simulink model "MSDRPrimaryLoop"  (R2021b)
settings: Solver=VariableStepAuto  StartTime=0.0  StopTime=250000  MaxStep=1  MinStep=0.01  RelTol=1e-3
undefined symbols (not defined in the file): a_f, A_free_PHX, a_g, A_h_PHX, beta, beta_t, bubbleGeneratorArea, bubbleGeneratorDh, bubbleGeneratorElevation, bubbleGeneratorLength, bubbleGeneratorVolume, bubbleSaturationLevel, bubbleSeparatorArea, bubbleSeparatorDiameter, bubbleSeparatorDo, bubbleSeparatorLength, bubbleSeparatorSlope, bypassRatio, C0, coreFlowArea, coreFuelVolume, coreLowerPlenumArea, coreLowerPlenumHydraulicDiameter, coreLowerPlenumLength, coreLowerPlenumVolume, coreUpperPlenumArea, coreUpperPlenumHydraulicDiameter, coreUpperPlenumLength, coreUpperPlenumVolume, coreVolume, cpGraphite, dissolusionRatio, dMin, dScale, dsmConst, DXeG, Fiss_factor, fuelChannelHydrualicDiameter, fuelChannelLength, fuelDepositRatio, fuelFraction, fuelGraphiteArea, fuelGraphiteHeatTransferCoefficient, gamma0, gamma1, gamma2, generatorDsm, graphiteKDiff, graphiteUnitCellThickness, initialIodineConcentration, InitialXeMolarConcentration, InjectionRatio, injectionRatio, iodineDecayConstant, IodineDecayConstant, iodineYield, kGraphite, kScale, Lam, lam ... (+59)
libraries: fl_lib x272, nesl_utility x105, SimscapeFluids_lib x24, slpidlib x1
(part 11 of 12)

== system MSDRPrimaryLoop/Reactor/CoreTH&Inerti/Core/CoreTH/CoreLinearNode3 ==
  note: Private model diameters are for MSDR only. These are based on the slab geometry and are not applicable to different reactor core design.
  note: Model with 1D simplified cylindrical quasi static heat transfer. Bi=0.26.
      | Refer to Nuclear Systems: 8.5.6. Or FHMT:5.5.2.
      | This is roughly ok for lumped analysis.
  GasRef : Inport
  2PModification : Subsystem  ReferencedSubsystem=TwoPhaseModification
      settings: PortSchema="{\"entries\":[{\"content\":{\"sides\":[{\"content\":{\"connectorIds\":[\"LConn1\"]},\"type\":\"ConnectorPlacement.EquallySpacedRectSide\",\"uuid\":\"7546b4b7-b669-49c8-8f27-f696391ea3ad\"},{\"content\":{\"connectorIds\":[\"RConn1\"],\"side\":\"RIGHT\"},\"type\":\"ConnectorPlacement.EquallySpacedRectSide\",\"uuid\":\"0e6176f2-177c-4327-bcfa-9a190fe9083f\"},{\"content\":{\"connectorIds\":[\"LConn2\",\"In1\"],\"side\":\"TOP\"},\"type\":\"ConnectorPlacement.EquallySpacedRectSide\",\"uuid\":\"16faf74c-4635-4009-a5b3-33dd03b625c6\"},{\"content\":{\"connectorIds\":[\"RConn2\"],\"side\":\"BOTTOM\"},\"type\":\"ConnectorPlacement.EquallySpacedRectSide\",\"uuid\":\"2081d73b-bb08-4ad9-b5c8-e48a4e9c4e20\"}]},\"type\":\"ConnectorPlacement.EquallySpacedConnector\",\"uuid\":\"243e4075-206b-4747-a8bc-b8f10d9a577f\"}],\"packageUris\":[\"http://schema.mathworks.com/mf0/Connector/R2020b\"],\"version\":\"1.0\"}"
  Conductive Heat Transfer1 : fl_lib/Thermal/Thermal Elements/Conductive Heat Transfer  area=CoreVolume/CoreLength*(1-FuelFraction) m^2  thickness=0.5*CoreLength/N_nodes m  th_cond=k_graphite W/(m*K)  T_specify=off  T_priority=None  T=0 K  T_nominal_specify=off  T_nominal_unit=K  T_nominal_value=1  Q_specify=off  Q_priority=None  Q=0 W  Q_nominal_specify=off  Q_nominal_unit=W  Q_nominal_value=1
  Conductive Heat Transfer2 : fl_lib/Thermal/Thermal Elements/Conductive Heat Transfer  area=CoreVolume/CoreLength*(1-FuelFraction) m^2  thickness=0.5*CoreLength/N_nodes m  th_cond=k_graphite W/(m*K)  T_specify=off  T_priority=None  T=0 K  T_nominal_specify=off  T_nominal_unit=K  T_nominal_value=1  Q_specify=off  Q_priority=None  Q=0 W  Q_nominal_specify=off  Q_nominal_unit=W  Q_nominal_value=1
  Conductive Heat Transfer3 : fl_lib/Thermal/Thermal Elements/Conductive Heat Transfer  area=FuelGraphiteArea/N_nodes m^2  thickness=0.5*UnitCellGraphiteThickness m  th_cond=k_graphite W/(m*K)  T_specify=off  T_priority=None  T=0 K  T_nominal_specify=off  T_nominal_unit=K  T_nominal_value=1  Q_specify=off  Q_priority=None  Q=0 W  Q_nominal_specify=off  Q_nominal_unit=W  Q_nominal_value=1
  Constant Volume Chamber (TL) : fl_lib/Thermal Liquid/Elements/Constant Volume Chamber (TL)  volume=0.001 m^3  num_ports=foundation.enum.num_ports.two  area_A=0.01 m^2  area_B=0.01 m^2  area_C=0.01 m^2  area_D=0.01 m^2  p_I_specify=on  p_I_priority=None  p_I=P0 Pa  p_I_nominal_specify=off  p_I_nominal_unit=MPa  p_I_nominal_value=1  T_I_specify=on  T_I_priority=None  T_I=T0 K  T_I_nominal_specify=off  T_I_nominal_unit=K  T_I_nominal_value=1  u_chamber_specify=on  u_chamber_priority=None  u_chamber=cpMSRE J/kg  u_chamber_nominal_specify=off  u_chamber_nominal_unit=kJ/kg  u_chamber_nominal_value=1  rho_specify=on  rho_priority=None  rho=nominalFuelDensity kg/m^3  rho_nominal_specify=off  rho_nominal_unit=kg/m^3  rho_nominal_value=1
      settings: SourceProductBaseCode=SS  LogSimulationData=on  InternalSimscapePortConfiguration="{\"Bottom\":[],\"Left\":[{\"id\":\"A\",\"label\":\"A\",\"type\":\"foundation.thermal_liquid.thermal_liquid\"},{\"id\":\"H\",\"label\":\"H\",\"type\":\"foundation.thermal.thermal\"}],\"Right\":[{\"id\":\"B\",\"label\":\"B\",\"type\":\"foundation.thermal_liquid.thermal_liquid\"}],\"Top\":[]}"
  Controlled Heat Flow Rate Source : fl_lib/Thermal/Thermal Sources/Controlled Heat Flow Rate Source
      settings: LogSimulationData=on
  Convective Heat Transfer : fl_lib/Thermal/Thermal Elements/Convective Heat Transfer  area=fuelGraphiteArea/N_nodes m^2  heat_tr_coeff=fuelGraphiteHeatTransferCoefficient W/(m^2*K)  T_specify=off  T_priority=None  T=0 K  T_nominal_specify=off  T_nominal_unit=K  T_nominal_value=1  Q_specify=off  Q_priority=None  Q=0 W  Q_nominal_specify=off  Q_nominal_unit=W  Q_nominal_value=1
  Fuel Deposited : fl_lib/Physical Signals/Functions/PS Gain  gain=FuelDepositRatio*CoreVolume/N_nodes m^3
  Grahite Deposited : fl_lib/Thermal/Thermal Sources/Controlled Heat Flow Rate Source
      settings: LogSimulationData=on
  Graphite Deposited : fl_lib/Physical Signals/Functions/PS Gain  gain=(1-FuelDepositRatio)*CoreVolume/N_nodes m^3
  Pipe (TL) : SimscapeFluids_lib/Thermal Liquid/Pipes & Fittings/Pipe (TL)  dynamic_compressibility=simscape.enum.onoff.on  inertia=simscape.enum.onoff.off  num_segments=1  pipe_length=fuelChannelLength/N_nodes m  area=coreFlowArea m^2  Dh=0.1128 m  wall_spec=fluids.thermal_liquid.pipes_fittings.enum.wall_spec.rigid  Dh_rigid=fuelChannelHydrualicDiameter m  wall_compliance=1.2e-6 m/MPa  wall_time_constant=0.01 s  elevation_spec=foundation.enum.constant_variable.constant  elevation_gain=fuelChannelLength/N_nodes m  g=9.82 m/s^2  pressure_loss_spec=fluids.thermal_liquid.pipes_fittings.enum.PressureLossSpec.Haaland  length_add=1 m  roughness=surfaceRoughness m  Re_friction_TLU=[400, 1000, 1500, 3000, 4000, 6000, 10000, 20000, 40000, 60000, 100000, 100000000]  friction_factor_TLU=[.264, .112, .071, .0417, .0387, .0268, .025, .0232, .0226, .022, .0214, .0214]  shape_factor=64  Re_lam=2000  Re_tur=4000  mdot_nominal=[.1, 1] kg/s  p_diff_nominal=[.001, .01] MPa  mdot_threshold=1e-6 kg/s  heat_transfer_spec=fluids.thermal_liquid.pipes_fittings.enum.HeatTransferSpec.Gnielinski  mdot_nominal_heat=[0.1, 10000] kg/s  T_in_nominal=[T0, T0] K  T_out_nominal=[T0, T0] K  p_in_nominal_heat=[.101325, .101325] MPa  T_wall_nominal=[T0+1, T0+1] K  a_coeff=0.023  b_Re_power=0.8  c_Pr_power=0.4  Nu_lam=3.66  Re_Colburn_TLU=[100, 150, 1000]  Colburn_factor_TLU=[.019, .013, .002]  Re_Nu_TLU=[100, 150, 1000]  Pr_Nu_TLU=[1, 10]  Nu_TLU=[3.72, 4.21; 3.75, 4.44; 4.21, 7.15]  T0_vec=T0 K  p0_vec=P0 Pa  mdot0=0.1 kg/s
      settings: SourceProductBaseCode=SH
  Temperature Sensor : fl_lib/Thermal/Thermal Sensors/Temperature Sensor
  Thermal Mass : fl_lib/Thermal/Thermal Elements/Thermal Mass  mass=CoreVolume*(1-FuelFraction)*rho_graphite/N_nodes kg  sp_heat=cp_graphite J/(K*kg)  T_specify=on  T_priority=High  T=T0 K  T_nominal_specify=off  T_nominal_unit=K  T_nominal_value=1  Q_specify=off  Q_priority=None  Q=0 W  Q_nominal_specify=off  Q_nominal_unit=W  Q_nominal_value=1
      settings: LogSimulationData=on
  Thermal Reference : fl_lib/Thermal/Thermal Elements/Thermal Reference
  Thermal Reference1 : fl_lib/Thermal/Thermal Elements/Thermal Reference
  Thermal Reference2 : fl_lib/Thermal/Thermal Elements/Thermal Reference
  Inlet : PMIOPort  Side=Left
  GraphiteA : PMIOPort  Port=2  Side=Left
  PowerDensity : PMIOPort  Port=3  Side=Left
  Outlet : PMIOPort  Port=4  Side=Right
  GraphiteB : PMIOPort  Port=5  Side=Right
  FuelTemp : PMIOPort  Port=6  Side=Right
  wires:
  GasRef/1 -> 2PModification/1
  connections:
  Grahite Deposited/LConn1 -- Conductive Heat Transfer3/RConn1 -- Conductive Heat Transfer2/RConn1 -- Thermal Mass/LConn1 -- Conductive Heat Transfer1/LConn1
  Graphite Deposited/LConn1 -- Fuel Deposited/LConn1 -- PowerDensity/RConn1
  Conductive Heat Transfer1/RConn1 -- GraphiteB/RConn1
  Grahite Deposited/RConn1 -- Graphite Deposited/RConn1
  GraphiteA/RConn1 -- Conductive Heat Transfer2/LConn1
  Controlled Heat Flow Rate Source/RConn2 -- Thermal Reference/LConn1
  Grahite Deposited/RConn2 -- Thermal Reference1/LConn1
  Fuel Deposited/RConn1 -- Controlled Heat Flow Rate Source/RConn1
  Outlet/RConn1 -- 2PModification/RConn1
  Temperature Sensor/RConn1 -- Thermal Reference2/LConn1
  Temperature Sensor/RConn2 -- FuelTemp/RConn1
  Inlet/RConn1 -- Constant Volume Chamber (TL)/LConn1
  Conductive Heat Transfer3/LConn1 -- Temperature Sensor/LConn1 -- Convective Heat Transfer/RConn1
  Constant Volume Chamber (TL)/LConn2 -- Convective Heat Transfer/LConn1 -- Controlled Heat Flow Rate Source/LConn1 -- Pipe (TL)/LConn2
  2PModification/RConn2 -- 2PModification/LConn1 -- Pipe (TL)/RConn1
  Constant Volume Chamber (TL)/RConn1 -- 2PModification/LConn2 -- Pipe (TL)/LConn1

== system MSDRPrimaryLoop/Reactor/CoreTH&Inerti/Core/CoreTH/PowerDensity ==
  note: This is a bit weird as the decay power is part of the total power.
      | I need to check the ratio of total power to decay power.
      | The 750MWth has to be refering to the...I don't know really.
  DecayFraction : Inport
  NeutronFraction : Inport  Port=2
  DecayPowerDensity : fl_lib/Physical Signals/Sources/PS Constant  constant=ReactorPower/CoreVolume*FuelInCoreRatio W/m^3
  PS Gain : fl_lib/Physical Signals/Functions/PS Gain  gain=3
  PS Min : fl_lib/Physical Signals/Nonlinear Operators/PS Min
      settings: SourceProductBaseCode=SS  InternalSimscapePortConfiguration="{\"Bottom\":[],\"Left\":[{\"id\":\"I1\",\"label\":\"\",\"type\":\"input\"},{\"id\":\"I2\",\"label\":\"\",\"type\":\"input\"}],\"Right\":[{\"id\":\"O\",\"label\":\"\",\"type\":\"output\"}],\"Top\":[]}"
  PS Product : fl_lib/Physical Signals/Functions/PS Product
  PS Product1 : fl_lib/Physical Signals/Functions/PS Product
  PowerDensity : fl_lib/Physical Signals/Sources/PS Constant  constant=ReactorPower/CoreVolume W/m^3
  Simulink-PS Converter : nesl_utility/Simulink-PS Converter  PhysicalDomain=network_engine_domain  SubClassName=ps_input  LeftPortType=input  RightPortType=output  PseudoPeriodic=off  Frequencies=[]  NoiseDistribution=none  NoiseParameters=[]  Unit=1  AffineConversion=off  FilteringAndDerivatives=provide  SimscapeFilterOrder=1  InputFilterTimeConstant=0.001  UdotUserProvided=0
      settings: SourceProductBaseCode=PW,SS
  Simulink-PS Converter1 : nesl_utility/Simulink-PS Converter  PhysicalDomain=network_engine_domain  SubClassName=ps_input  LeftPortType=input  RightPortType=output  PseudoPeriodic=off  Frequencies=[]  NoiseDistribution=none  NoiseParameters=[]  Unit=1  AffineConversion=off  FilteringAndDerivatives=provide  SimscapeFilterOrder=1  InputFilterTimeConstant=0.001  UdotUserProvided=0
      settings: SourceProductBaseCode=PW,SS
  TotalCorePower : fl_lib/Physical Signals/Functions/PS Add
  Conn1 : PMIOPort  Side=Right
  wires:
  DecayFraction/1 -> Simulink-PS Converter1/1
  NeutronFraction/1 -> Simulink-PS Converter/1
  connections:
  PS Product/RConn1 -- TotalCorePower/LConn1
  TotalCorePower/RConn1 -- PS Min/LConn2
  DecayPowerDensity/RConn1 -- PS Product1/LConn2
  PS Gain/RConn1 -- PS Min/LConn1
  Simulink-PS Converter/RConn1 -- PS Product/LConn2
  Simulink-PS Converter1/RConn1 -- PS Product1/LConn1
  PS Product1/RConn1 -- TotalCorePower/LConn2
  PS Min/RConn1 -- Conn1/RConn1
  PS Product/LConn1 -- PowerDensity/RConn1 -- PS Gain/LConn1

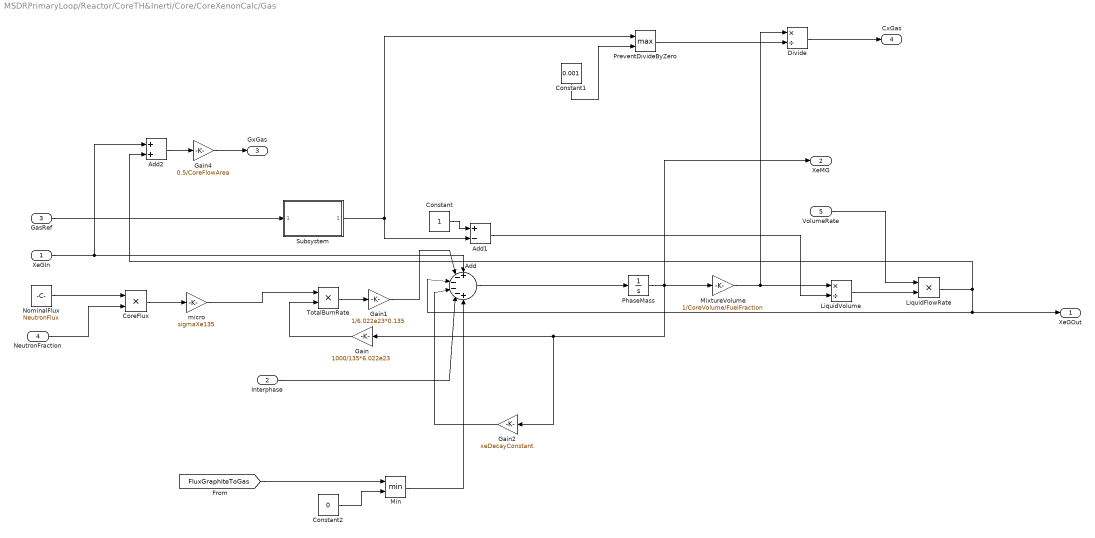
== system MSDRPrimaryLoop/Reactor/CoreTH&Inerti/Core/CoreXenonCalc/Gas ==
  XeGIn : Inport
  Interphase : Inport  Port=2
  GasRef : Inport  Port=3
  NeutronFraction : Inport  Port=4
  VolumeRate : Inport  Port=5
  Add : Sum  Inputs=+----+
  Add1 : Sum  Inputs=+-
  Add2 : Sum
  Constant : Constant
  Constant1 : Constant  Value=0.001
  Constant2 : Constant  Value=0
  CoreFlux : Product
  Divide : Product  Inputs=*/
  Gain : Gain  Gain=1000/135*6.022e23
  Gain1 : Gain  Gain=1/6.022e23*0.135
  Gain2 : Gain  Gain=xeDecayConstant
  Gain4 : Gain  Gain=0.5/CoreFlowArea
  LiquidFlowRate : Product
  LiquidVolume : Product  Inputs=*/
  Min : MinMax  Inputs=2
  MixtureVolume : Gain  Gain=1/CoreVolume/FuelFraction
  NominalFlux : Constant  Value=NeutronFlux
  PhaseMass : Integrator  LimitOutput=on  LowerSaturationLimit=0
  PreventDivideByZero : MinMax  Function=max  Inputs=2
  Subsystem : Subsystem  ReferencedSubsystem=GasToAlpha
  TotalBurnRate : Product
  micro : Gain  Gain=sigmaXe135
  XeGOut : Outport
  XeMG : Outport  Port=2
  GxGas : Outport  Port=3
  CxGas : Outport  Port=4
  wires:
  LiquidFlowRate/1 -> XeGOut/1, Add/3, Add2/2
  NominalFlux/1 -> CoreFlux/1
  LiquidVolume/1 -> LiquidFlowRate/2
  Add/1 -> PhaseMass/1
  CoreFlux/1 -> micro/1
  NeutronFraction/1 -> CoreFlux/2
  Constant/1 -> Add1/1
  Add1/1 -> LiquidVolume/2
  VolumeRate/1 -> LiquidFlowRate/1
  GasRef/1 -> Subsystem/1
  XeGIn/1 -> Add2/1, Add/1
  micro/1 -> TotalBurnRate/1
  Gain/1 -> TotalBurnRate/2
  TotalBurnRate/1 -> Gain1/1
  Gain1/1 -> Add/2
  Gain2/1 -> Add/4
  PhaseMass/1 -> XeMG/1, Gain2/1, Gain/1, MixtureVolume/1
  Interphase/1 -> Add/5
  Gain4/1 -> GxGas/1
  Add2/1 -> Gain4/1
  Constant1/1 -> PreventDivideByZero/2
  Divide/1 -> CxGas/1
  PreventDivideByZero/1 -> Divide/2
  MixtureVolume/1 -> LiquidVolume/1, Divide/1
  Subsystem/1 -> PreventDivideByZero/1, Add1/2
  [FluxGraphiteToGas] -> Min/1
  Min/1 -> Add/6
  Constant2/1 -> Min/2

== system MSDRPrimaryLoop/Reactor/CoreTH&Inerti/Core/CoreXenonCalc/InterphaseTranfser ==
  GxSalt : Inport
  NeutronFraction : Inport  Port=2
  GasRef : Inport  Port=3
  GxGas : Inport  Port=4
  CxSalt : Inport  Port=5
  T_f_ave : Inport  Port=6
  PLoss : Inport  Port=7
  CxGas : Inport  Port=8
  VolumeRate : Inport  Port=9
  Constant : Constant  Value=Dh
  Constant1 : Constant  Value=nominalNeutronFlux
  Constitutive : Subsystem
      settings: PortSchema="{\"entries\":[{\"content\":{\"sides\":[{\"content\":{\"connectorIds\":[\"In1\",\"LConn1\",\"In2\",\"In3\",\"In4\"]},\"type\":\"ConnectorPlacement.EquallySpacedRectSide\",\"uuid\":\"b30af6c3-7c55-4661-bc76-939f1c8a4177\"},{\"content\":{\"connectorIds\":[\"Out1\",\"Out2\",\"Out3\",\"Out4\",\"Out5\",\"Out6\",\"Out7\",\"Out8\",\"Out9\"],\"side\":\"RIGHT\"},\"type\":\"ConnectorPlacement.EquallySpacedRectSide\",\"uuid\":\"0b137634-5e01-4bd6-8381-72b0699f5835\"},{\"content\":{\"connectorIds\":[],\"side\":\"TOP\"},\"type\":\"ConnectorPlacement.EquallySpacedRectSide\",\"uuid\":\"06046061-3240-493e-a0a3-282c9541adae\"}]},\"type\":\"ConnectorPlacement.EquallySpacedConnector\",\"uuid\":\"b0591291-fd4b-4355-beaa-e569a19c4b12\"}],\"packageUris\":[\"http://schema.mathworks.com/mf0/Connector/R2020b\"],\"version\":\"1.0\"}"
  GraphiteInterchangeModel : Subsystem  mask{FuelGraphiteArea=FuelGraphiteArea, GraphiteVolume=CoreVolume*(1-FuelFraction), GraphitePorosity=0.1}
      mask prompts: FuelGraphiteArea "Fuel-Graphite Interface Area"; GraphiteVolume "Graphite Volume"; GraphitePorosity "Graphite Porosity"
  MixtureVolume : Gain  Gain=CoreVolume*FuelFraction
  Product : Product
  String Constant : StringConstant  String="\"upwards\""
  Subsystem : Subsystem  ReferencedSubsystem=kCalculation
      settings: PortSchema="{\"entries\":[{\"content\":{\"sides\":[{\"content\":{\"connectorIds\":[\"In2\",\"In3\",\"In4\",\"In5\",\"In6\",\"In7\",\"In1\"]},\"type\":\"ConnectorPlacement.EquallySpacedRectSide\",\"uuid\":\"002a6616-4b3b-4d3e-9efd-a784f6bbe134\"},{\"content\":{\"connectorIds\":[\"Out1\",\"Out2\"],\"side\":\"RIGHT\"},\"type\":\"ConnectorPlacement.EquallySpacedRectSide\",\"uuid\":\"da6acc14-6515-461b-8149-f4cbf493a4dd\"},{\"content\":{\"connectorIds\":[],\"side\":\"TOP\"},\"type\":\"ConnectorPlacement.EquallySpacedRectSide\",\"uuid\":\"939e49a4-f3cd-4ed3-a7a5-6bbefe0ae08a\"},{\"content\":{\"connectorIds\":[\"In8\"],\"side\":\"BOTTOM\"},\"type\":\"ConnectorPlacement.EquallySpacedRectSide\",\"uuid\":\"1ce110d7-af97-437a-ade8-04ae9fcd8383\"}]},\"type\":\"ConnectorPlacement.EquallySpacedConnector\",\"uuid\":\"8f0c794e-eb76-47c6-abaf-8e07cad1f307\"}],\"packageUris\":[\"http://schema.mathworks.com/mf0/Connector/R2020b\"],\"version\":\"1.0\"}"
  Subsystem1 : Subsystem  ReferencedSubsystem=GasToAlpha
  Transfer Term : MATLAB Function  TreatAsAtomicUnit=on
  Ref : PMIOPort  Side=Left
  TranfserRate : Outport
  XeMGraphite : Outport  Port=2
  tag scope: FluxGraphiteToGas=global, FluxGraphiteToSalt=global
  wires:
  Transfer Term/1(volRate) -> MixtureVolume/1
  MixtureVolume/1 -> TranfserRate/1
  Subsystem/2 -> Transfer Term/8(k)
  Subsystem/1 -> GraphiteInterchangeModel/5(dsm), Transfer Term/7(dsm)
  VolumeRate/1 -> Constitutive/3(VolumeRate)
  GasRef/1 -> Subsystem1/1
  Subsystem1/1 -> Constitutive/1(alpha), Transfer Term/3(alpha), GraphiteInterchangeModel/6(GasRef)
  Constitutive/1(ul) -> Transfer Term/4(ul), GraphiteInterchangeModel/7(ul)
  Constitutive/2(ug) -> Transfer Term/5(ug)
  Constitutive/3(K) -> Transfer Term/6(K)
  Constant/1 -> Subsystem/7, Constitutive/4(Diam)
  GxSalt/1 -> Transfer Term/1(GxS)
  GxGas/1 -> Transfer Term/2(GxG)
  CxGas/1 -> GraphiteInterchangeModel/4(CXeg)
  CxSalt/1 -> GraphiteInterchangeModel/1(CXef)
  T_f_ave/1 -> GraphiteInterchangeModel/3(Tempature)
  GraphiteInterchangeModel/3(Gas Diffusion Rate) -> [FluxGraphiteToGas]
  GraphiteInterchangeModel/1(Salt Diffusion Rate) -> [FluxGraphiteToSalt]
  GraphiteInterchangeModel/2(Xenon Mass In Graphite) -> XeMGraphite/1
  PLoss/1 -> Constitutive/2(PLoss)
  Constitutive/4(Re) -> Subsystem/2
  Constitutive/5(Sc) -> Subsystem/3
  Constitutive/6(Diff) -> Subsystem/4
  Constitutive/7(alphaC) -> Subsystem/5
  Constitutive/8(dsm) -> Subsystem/6
  Constitutive/9(f_m) -> Subsystem/1
  Constant1/1 -> Product/1
  NeutronFraction/1 -> Product/2
  Product/1 -> GraphiteInterchangeModel/2(phi)
  String Constant/1 -> Subsystem/8
  connections:
  Constitutive/LConn1 -- Ref/RConn1

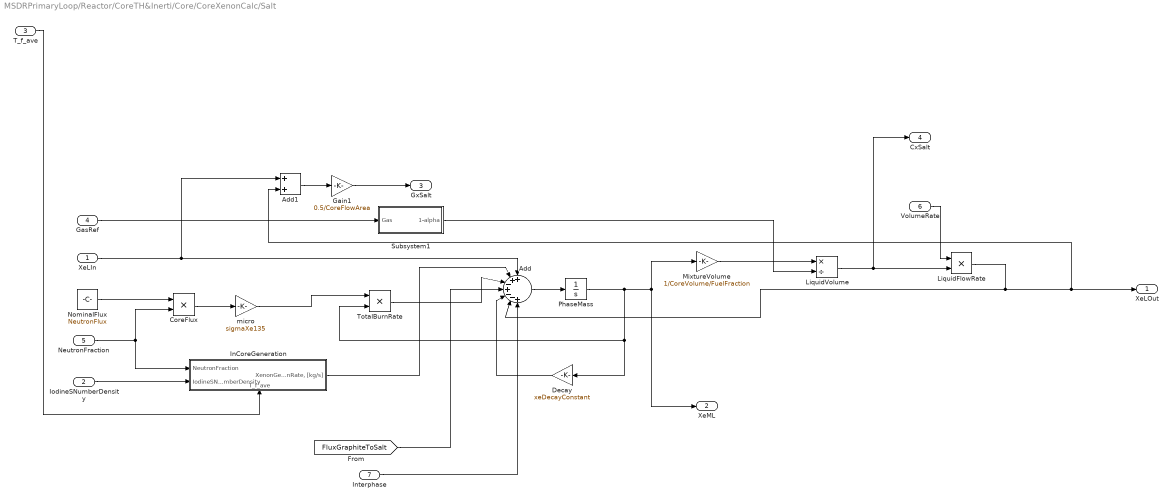
== system MSDRPrimaryLoop/Reactor/CoreTH&Inerti/Core/CoreXenonCalc/Salt ==
  XeLIn : Inport  PortDimensions=1
  IodineSNumberDensity : Inport  Port=2  PortDimensions=1
  T_f_ave : Inport  Port=3
  GasRef : Inport  Port=4  PortDimensions=1
  NeutronFraction : Inport  Port=5  PortDimensions=1
  VolumeRate : Inport  Port=6
  Interphase : Inport  Port=7
  Add : Sum  Inputs=++-+--+  InputSameDT=on
  Add1 : Sum
  CoreFlux : Product
  Decay : Gain  Gain=xeDecayConstant
  Gain1 : Gain  Gain=0.5/CoreFlowArea
  InCoreGeneration : Subsystem
      settings: PortSchema="{\"entries\":[{\"content\":{\"sides\":[{\"content\":{\"connectorIds\":[\"In1\",\"In2\"]},\"type\":\"ConnectorPlacement.EquallySpacedRectSide\",\"uuid\":\"cf58f9e2-4051-4ec0-bfd5-a375f3464f67\"},{\"content\":{\"connectorIds\":[\"Out1\"],\"side\":\"RIGHT\"},\"type\":\"ConnectorPlacement.EquallySpacedRectSide\",\"uuid\":\"cf475b22-0422-4ebc-b148-ab559744c6ba\"},{\"content\":{\"connectorIds\":[],\"side\":\"TOP\"},\"type\":\"ConnectorPlacement.EquallySpacedRectSide\",\"uuid\":\"15cc78ce-ee79-4f49-b098-b77c0b2a8ba1\"},{\"content\":{\"connectorIds\":[\"In3\"],\"side\":\"BOTTOM\"},\"type\":\"ConnectorPlacement.EquallySpacedRectSide\",\"uuid\":\"64f5be1f-19d6-4b5f-ac24-c41659a6a539\"}]},\"type\":\"ConnectorPlacement.EquallySpacedConnector\",\"uuid\":\"1fb1607a-ceed-4d70-a511-7b706be0d7ea\"}],\"packageUris\":[\"http://schema.mathworks.com/mf0/Connector/R2020b\"],\"version\":\"1.0\"}"
  LiquidFlowRate : Product
  LiquidVolume : Product  Inputs=*/
  MixtureVolume : Gain  Gain=1/CoreVolume/FuelFraction
  NominalFlux : Constant  Value=NeutronFlux
  PhaseMass : Integrator  LimitOutput=on  LowerSaturationLimit=0
  Subsystem1 : Subsystem
  TotalBurnRate : Product
  micro : Gain  Gain=sigmaXe135
  XeLOut : Outport  PortDimensions=1
  XeML : Outport  Port=2  PortDimensions=1
  GxSalt : Outport  Port=3
  CxSalt : Outport  Port=4
  wires:
  LiquidFlowRate/1 -> Add/6, Add1/2, XeLOut/1
  IodineSNumberDensity/1 -> InCoreGeneration/2(IodineSNumberDensity)
  NominalFlux/1 -> CoreFlux/1
  LiquidVolume/1 -> CxSalt/1, LiquidFlowRate/2
  Add/1 -> PhaseMass/1
  CoreFlux/1 -> micro/1
  NeutronFraction/1 -> InCoreGeneration/1(NeutronFraction), CoreFlux/2
  MixtureVolume/1 -> LiquidVolume/1
  VolumeRate/1 -> LiquidFlowRate/1
  T_f_ave/1 -> InCoreGeneration/3(T_f_ave)
  XeLIn/1 -> Add1/1, Add/1
  micro/1 -> TotalBurnRate/1
  PhaseMass/1 -> TotalBurnRate/2, Decay/1, XeML/1, MixtureVolume/1
  Decay/1 -> Add/5
  GasRef/1 -> Subsystem1/1(Gas)
  Subsystem1/1(1-alpha) -> LiquidVolume/2
  [FluxGraphiteToSalt] -> Add/4
  InCoreGeneration/1("XenonGenerationRate, [kg/s]") -> Add/2
  TotalBurnRate/1 -> Add/3
  Interphase/1 -> Add/7
  Gain1/1 -> GxSalt/1
  Add1/1 -> Gain1/1

== system MSDRPrimaryLoop/Reactor/CoreTH&Inerti/Core/SolubilityReduction/If Action Subsystem ==
  GasLeft : Inport
  Action Port : ActionPort  ActionPortLabel=if(u1 > 0)
  Constant : Constant  Value=dissolusionRatio
  Gain : Gain
  GasOut : Outport
  AbsorbedGas : Outport  Port=2
  wires:
  GasLeft/1 -> GasOut/1
  Constant/1 -> Gain/1
  Gain/1 -> AbsorbedGas/1

== system MSDRPrimaryLoop/Reactor/CoreTH&Inerti/Core/SolubilityReduction/If Action Subsystem1 ==
  GasIn : Inport
  Action Port : ActionPort  ActionPortLabel=else
  Constant : Constant  Value=0
  GasOut : Outport
  AbsorbedGas : Outport  Port=2
  wires:
  GasIn/1 -> AbsorbedGas/1
  Constant/1 -> GasOut/1

== system MSDRPrimaryLoop/Reactor/CoreTH&Inerti/Core/Subsystem1/GasCalc ==
  GasIn : Inport
  Add : Sum  Inputs=+-
  GasExpansion : Subsystem  ReferencedSubsystem=GasExpansion
      settings: PortSchema="{\"entries\":[{\"content\":{\"sides\":[{\"content\":{\"connectorIds\":[\"LConn1\",\"In1\"]},\"type\":\"ConnectorPlacement.EquallySpacedRectSide\",\"uuid\":\"50c89675-cb8a-4964-af62-cb2014507b1d\"},{\"content\":{\"connectorIds\":[\"RConn1\",\"Out1\"],\"side\":\"RIGHT\"},\"type\":\"ConnectorPlacement.EquallySpacedRectSide\",\"uuid\":\"6b3adc78-0be5-4682-9da0-6fd41ffc4e71\"},{\"content\":{\"connectorIds\":[],\"side\":\"TOP\"},\"type\":\"ConnectorPlacement.EquallySpacedRectSide\",\"uuid\":\"5158b46f-a496-48e4-90d6-6c6dcc9e237b\"}]},\"type\":\"ConnectorPlacement.EquallySpacedConnector\",\"uuid\":\"7ff0188e-dc19-44a0-a8cf-bde33949414f\"}],\"packageUris\":[\"http://schema.mathworks.com/mf0/Connector/R2020b\"],\"version\":\"1.0\"}"
  Integrator : Integrator  InitialCondition=injectionRatio*CoreVolume*FuelFraction
  PS-Simulink Converter : nesl_utility/PS-Simulink Converter  PhysicalDomain=network_engine_domain  SubClassName=ps_output  LeftPortType=input  RightPortType=output  PseudoPeriodic=off  Frequencies=[]  Unit=inherit  AffineConversion=off
      settings: SourceProductBaseCode=PW,SS
  Product : Product
  VolumeToVoid : Gain  Gain=1/(CoreVolume*FuelFraction)
  VolumeRate : PMIOPort  Side=Left
  Ref1 : PMIOPort  Port=2  Side=Right
  Ref2 : PMIOPort  Port=3  Side=Right
  GasOut : Outport
  wires:
  VolumeToVoid/1 -> GasExpansion/1, Add/2
  Integrator/1 -> VolumeToVoid/1
  GasIn/1 -> Add/1
  Add/1 -> Product/1
  Product/1 -> Integrator/1
  PS-Simulink Converter/1 -> Product/2
  GasExpansion/1 -> GasOut/1
  connections:
  PS-Simulink Converter/LConn1 -- VolumeRate/RConn1
  GasExpansion/LConn1 -- Ref1/RConn1
  GasExpansion/RConn1 -- Ref2/RConn1

== system MSDRPrimaryLoop/Reactor/CoreTH&Inerti/Core/Subsystem2/SolubilityModificationPrescribed ==
  note: The idea is that when the dissolved gas comes back out, it is saturated with xenon because of the super efficiency removal of micro bubbles. The gain factor is used to adjust the concentration of the bubbles to less than saturation.
  XeIn : Inport
  GasIn : Inport  Port=2
  AbsorbedOut : Inport  Port=3
  Temperature : Inport  Port=4
  Add : Sum
  Add1 : Sum
  AddedBackGas : Sum
  Constant : Constant
  Demux : Demux  Outputs=2
  Divide : Product  Inputs=**/
  Divide1 : Product  Inputs=*/
  Divide2 : Product  Inputs=*/
  Gain : Gain  Gain=bubbleSaturationLevel
  KScale : Subsystem  ReferencedSubsystem=KScale
  Mux : Mux  Inputs=2
  XeOut : Outport
  GasOut : Outport  Port=2
  wires:
  GasIn/1 -> AddedBackGas/1
  AbsorbedOut/1 -> Divide2/1, AddedBackGas/2
  AddedBackGas/1 -> GasOut/1
  XeIn/1 -> Demux/1
  Mux/1 -> XeOut/1
  Temperature/1 -> KScale/1
  KScale/1 -> Divide2/2
  Constant/1 -> Add/2
  Divide2/1 -> Gain/1
  Add/1 -> Divide1/2, Divide/3
  Demux/1 -> Divide/1, Divide1/1
  Demux/2 -> Add1/1
  Divide/1 -> Add1/2
  Add1/1 -> Mux/2
  Divide1/1 -> Mux/1
  Gain/1 -> Add/1, Divide/2

== system MSDRPrimaryLoop/Reactor/CoreTH&Inerti/Core/Subsystem2/Subsystem2 ==
  note: Switch between prescibed concentration and near-zero based on whether bubbles are present.
  XeIn : Inport
  GasIn : Inport  Port=2
  AbsorbedOut : Inport  Port=3
  Temperature : Inport  Port=4
  ModeSwitch : Inport  Port=5
  If : If
  If Action Subsystem : Subsystem  TreatAsAtomicUnit=on
  If Action Subsystem1 : Subsystem  TreatAsAtomicUnit=on
  Merge : Merge
  Merge1 : Merge
  GasOut : Outport
  XeOut : Outport  Port=2
  wires:
  ModeSwitch/1 -> If/1
  If/1 -> If Action Subsystem/Action
  If/2 -> If Action Subsystem1/Action
  AbsorbedOut/1 -> If Action Subsystem1/2(AbsorbedOut), If Action Subsystem/2(AbsorbedOut)
  GasIn/1 -> If Action Subsystem1/1(GasIn), If Action Subsystem/1(GasIn)
  XeIn/1 -> If Action Subsystem/3(XeIn), If Action Subsystem1/3(XeIn)
  Merge/1 -> GasOut/1
  If Action Subsystem/1(GasOut) -> Merge/1
  If Action Subsystem1/1(GasOut) -> Merge/2
  If Action Subsystem/2(XeOut) -> Merge1/1
  If Action Subsystem1/2(XeOut) -> Merge1/2
  Merge1/1 -> XeOut/1
  Temperature/1 -> If Action Subsystem1/4(Temperature)

== system MSDRPrimaryLoop/Reactor/CoreTH&Inerti/LowerPlenum/XenonCalc/Gas ==
  XeGIn : Inport
  Interphase : Inport  Port=2
  GasRef : Inport  Port=3
  VolumeRate : Inport  Port=4
  Add : Sum  Inputs=+---
  Add1 : Sum  Inputs=+-
  Add2 : Sum
  Constant : Constant
  Gain2 : Gain  Gain=xeDecayConstant
  Gain4 : Gain  Gain=0.5/Area
  LiquidFlowRate : Product
  LiquidVolume : Product  Inputs=*/
  MixtureVolume : Gain  Gain=1/Volume
  PhaseMass : Integrator  LimitOutput=on  LowerSaturationLimit=0
  Subsystem : Subsystem  ReferencedSubsystem=GasToAlpha
  XeGOut : Outport
  GxGas : Outport  Port=2
  wires:
  LiquidFlowRate/1 -> XeGOut/1, Add2/2, Add/3
  Subsystem/1 -> Add1/2
  LiquidVolume/1 -> LiquidFlowRate/2
  Add/1 -> PhaseMass/1
  Constant/1 -> Add1/1
  MixtureVolume/1 -> LiquidVolume/1
  Add1/1 -> LiquidVolume/2
  VolumeRate/1 -> LiquidFlowRate/1
  GasRef/1 -> Subsystem/1
  XeGIn/1 -> Add/1, Add2/1
  Gain2/1 -> Add/4
  PhaseMass/1 -> Gain2/1, MixtureVolume/1
  Gain4/1 -> GxGas/1
  Add2/1 -> Gain4/1
  Interphase/1 -> Add/2

== system MSDRPrimaryLoop/Reactor/CoreTH&Inerti/LowerPlenum/XenonCalc/InterphaseTranfser ==
  note: This local to volume isn't strick. Either add an integral or reduce the length of the node if variation is large.
  GxSalt : Inport
  GasRef : Inport  Port=2
  GxGas : Inport  Port=3
  PLoss : Inport  Port=4
  VolumeRate : Inport  Port=5
  Constant : Constant  Value=Dh
  Constitutive : Subsystem
      settings: PortSchema="{\"entries\":[{\"content\":{\"sides\":[{\"content\":{\"connectorIds\":[\"In1\",\"LConn1\",\"In2\",\"In3\",\"In4\"]},\"type\":\"ConnectorPlacement.EquallySpacedRectSide\",\"uuid\":\"b30af6c3-7c55-4661-bc76-939f1c8a4177\"},{\"content\":{\"connectorIds\":[\"Out1\",\"Out2\",\"Out3\",\"Out4\",\"Out5\",\"Out6\",\"Out7\",\"Out8\",\"Out9\"],\"side\":\"RIGHT\"},\"type\":\"ConnectorPlacement.EquallySpacedRectSide\",\"uuid\":\"0b137634-5e01-4bd6-8381-72b0699f5835\"},{\"content\":{\"connectorIds\":[],\"side\":\"TOP\"},\"type\":\"ConnectorPlacement.EquallySpacedRectSide\",\"uuid\":\"06046061-3240-493e-a0a3-282c9541adae\"}]},\"type\":\"ConnectorPlacement.EquallySpacedConnector\",\"uuid\":\"b0591291-fd4b-4355-beaa-e569a19c4b12\"}],\"packageUris\":[\"http://schema.mathworks.com/mf0/Connector/R2020b\"],\"version\":\"1.0\"}"
  MixtureVolume : Gain  Gain=Volume
  String Constant : StringConstant  String="\"upwards\""
  Subsystem : Subsystem  ReferencedSubsystem=kCalculation
      settings: PortSchema="{\"entries\":[{\"content\":{\"sides\":[{\"content\":{\"connectorIds\":[\"In2\",\"In3\",\"In4\",\"In5\",\"In6\",\"In7\",\"In1\"]},\"type\":\"ConnectorPlacement.EquallySpacedRectSide\",\"uuid\":\"002a6616-4b3b-4d3e-9efd-a784f6bbe134\"},{\"content\":{\"connectorIds\":[\"Out1\",\"Out2\"],\"side\":\"RIGHT\"},\"type\":\"ConnectorPlacement.EquallySpacedRectSide\",\"uuid\":\"da6acc14-6515-461b-8149-f4cbf493a4dd\"},{\"content\":{\"connectorIds\":[],\"side\":\"TOP\"},\"type\":\"ConnectorPlacement.EquallySpacedRectSide\",\"uuid\":\"939e49a4-f3cd-4ed3-a7a5-6bbefe0ae08a\"},{\"content\":{\"connectorIds\":[\"In8\"],\"side\":\"BOTTOM\"},\"type\":\"ConnectorPlacement.EquallySpacedRectSide\",\"uuid\":\"df8afac6-b18f-4ec8-9e08-eea5226bf274\"}]},\"type\":\"ConnectorPlacement.EquallySpacedConnector\",\"uuid\":\"8f0c794e-eb76-47c6-abaf-8e07cad1f307\"}],\"packageUris\":[\"http://schema.mathworks.com/mf0/Connector/R2020b\"],\"version\":\"1.0\"}"
  Subsystem1 : Subsystem  ReferencedSubsystem=GasToAlpha
  Transfer Term : MATLAB Function  TreatAsAtomicUnit=on
  Ref : PMIOPort  Side=Left
  TranfserRate : Outport
  wires:
  Transfer Term/1(volRate) -> MixtureVolume/1
  MixtureVolume/1 -> TranfserRate/1
  VolumeRate/1 -> Constitutive/3(VolumeRate)
  GasRef/1 -> Subsystem1/1
  Subsystem1/1 -> Constitutive/1(alpha), Transfer Term/3(alpha)
  Constitutive/1(ul) -> Transfer Term/4(ul)
  Constitutive/2(ug) -> Transfer Term/5(ug)
  Constitutive/3(K) -> Transfer Term/6(K)
  Constant/1 -> Subsystem/7, Constitutive/4(Diam)
  GxSalt/1 -> Transfer Term/1(GxS)
  GxGas/1 -> Transfer Term/2(GxG)
  Constitutive/9(f_m) -> Subsystem/1
  Constitutive/4(Re) -> Subsystem/2
  Constitutive/5(Sc) -> Subsystem/3
  Constitutive/7(alphaC) -> Subsystem/5
  Subsystem/1 -> Transfer Term/7(dsm)
  Subsystem/2 -> Transfer Term/8(k)
  PLoss/1 -> Constitutive/2(PLoss)
  Constitutive/8(dsm) -> Subsystem/6
  Constitutive/6(Diff) -> Subsystem/4
  String Constant/1 -> Subsystem/8
  connections:
  Ref/RConn1 -- Constitutive/LConn1

== system MSDRPrimaryLoop/Reactor/CoreTH&Inerti/LowerPlenum/XenonCalc/Salt ==
  XeLIn : Inport  PortDimensions=1
  IodineSNumberDensity : Inport  Port=2  PortDimensions=1
  T_f_ave : Inport  Port=3
  GasRef : Inport  Port=4  PortDimensions=1
  VolumeRate : Inport  Port=5
  Interphase : Inport  Port=6
  Add : Sum  Inputs=+++--  InputSameDT=on
  Add1 : Sum
  Decay : Gain  Gain=xeDecayConstant
  Gain1 : Gain  Gain=0.5/Area
  InPipeGeneration : Subsystem
      settings: PortSchema="{\"entries\":[{\"content\":{\"sides\":[{\"content\":{\"connectorIds\":[\"In1\"]},\"type\":\"ConnectorPlacement.EquallySpacedRectSide\",\"uuid\":\"cf58f9e2-4051-4ec0-bfd5-a375f3464f67\"},{\"content\":{\"connectorIds\":[\"Out1\"],\"side\":\"RIGHT\"},\"type\":\"ConnectorPlacement.EquallySpacedRectSide\",\"uuid\":\"cf475b22-0422-4ebc-b148-ab559744c6ba\"},{\"content\":{\"connectorIds\":[],\"side\":\"TOP\"},\"type\":\"ConnectorPlacement.EquallySpacedRectSide\",\"uuid\":\"15cc78ce-ee79-4f49-b098-b77c0b2a8ba1\"},{\"content\":{\"connectorIds\":[\"In2\"],\"side\":\"BOTTOM\"},\"type\":\"ConnectorPlacement.EquallySpacedRectSide\",\"uuid\":\"64f5be1f-19d6-4b5f-ac24-c41659a6a539\"}]},\"type\":\"ConnectorPlacement.EquallySpacedConnector\",\"uuid\":\"1fb1607a-ceed-4d70-a511-7b706be0d7ea\"}],\"packageUris\":[\"http://schema.mathworks.com/mf0/Connector/R2020b\"],\"version\":\"1.0\"}"
  LiquidFlowRate : Product
  LiquidVolume : Product  Inputs=*/
  MixtureVolume : Gain  Gain=1/Volume
  PhaseMass : Integrator  LimitOutput=on  LowerSaturationLimit=0
  Subsystem1 : Subsystem
  XeLOut : Outport  PortDimensions=1
  GxSalt : Outport  Port=2
  wires:
  LiquidFlowRate/1 -> Add/5, XeLOut/1, Add1/2
  IodineSNumberDensity/1 -> InPipeGeneration/1(IodineSNumberDensity)
  LiquidVolume/1 -> LiquidFlowRate/2
  Add/1 -> PhaseMass/1
  MixtureVolume/1 -> LiquidVolume/1
  VolumeRate/1 -> LiquidFlowRate/1
  T_f_ave/1 -> InPipeGeneration/2(T_f_ave)
  PhaseMass/1 -> Decay/1, MixtureVolume/1
  GasRef/1 -> Subsystem1/1(Gas)
  Subsystem1/1(1-alpha) -> LiquidVolume/2
  InPipeGeneration/1("XenonGenerationRate, [kg/s]") -> Add/2
  XeLIn/1 -> Add1/1, Add/1
  Add1/1 -> Gain1/1
  Gain1/1 -> GxSalt/1
  Interphase/1 -> Add/3
  Decay/1 -> Add/4

== system MSDRPrimaryLoop/Reactor/CoreTH&Inerti/UpperPlenum/XenonCalc/Gas ==
  XeGIn : Inport
  Interphase : Inport  Port=2
  GasRef : Inport  Port=3
  VolumeRate : Inport  Port=4
  Add : Sum  Inputs=+---
  Add1 : Sum  Inputs=+-
  Add2 : Sum
  Constant : Constant
  Gain2 : Gain  Gain=xeDecayConstant
  Gain4 : Gain  Gain=0.5/Area
  LiquidFlowRate : Product
  LiquidVolume : Product  Inputs=*/
  MixtureVolume : Gain  Gain=1/Volume
  PhaseMass : Integrator  LimitOutput=on  LowerSaturationLimit=0
  Subsystem : Subsystem  ReferencedSubsystem=GasToAlpha
  XeGOut : Outport
  GxGas : Outport  Port=2
  wires:
  LiquidFlowRate/1 -> XeGOut/1, Add2/2, Add/3
  Subsystem/1 -> Add1/2
  LiquidVolume/1 -> LiquidFlowRate/2
  Add/1 -> PhaseMass/1
  Constant/1 -> Add1/1
  MixtureVolume/1 -> LiquidVolume/1
  Add1/1 -> LiquidVolume/2
  VolumeRate/1 -> LiquidFlowRate/1
  GasRef/1 -> Subsystem/1
  XeGIn/1 -> Add/1, Add2/1
  Gain2/1 -> Add/4
  PhaseMass/1 -> Gain2/1, MixtureVolume/1
  Gain4/1 -> GxGas/1
  Add2/1 -> Gain4/1
  Interphase/1 -> Add/2

== system MSDRPrimaryLoop/Reactor/CoreTH&Inerti/UpperPlenum/XenonCalc/InterphaseTranfser ==
  note: This local to volume isn't strick. Either add an integral or reduce the length of the node if variation is large.
  GxSalt : Inport
  GasRef : Inport  Port=2
  GxGas : Inport  Port=3
  PLoss : Inport  Port=4
  VolumeRate : Inport  Port=5
  Constant : Constant  Value=Dh
  Constitutive : Subsystem
      settings: PortSchema="{\"entries\":[{\"content\":{\"sides\":[{\"content\":{\"connectorIds\":[\"In1\",\"LConn1\",\"In2\",\"In3\",\"In4\"]},\"type\":\"ConnectorPlacement.EquallySpacedRectSide\",\"uuid\":\"b30af6c3-7c55-4661-bc76-939f1c8a4177\"},{\"content\":{\"connectorIds\":[\"Out1\",\"Out2\",\"Out3\",\"Out4\",\"Out5\",\"Out6\",\"Out7\",\"Out8\",\"Out9\"],\"side\":\"RIGHT\"},\"type\":\"ConnectorPlacement.EquallySpacedRectSide\",\"uuid\":\"0b137634-5e01-4bd6-8381-72b0699f5835\"},{\"content\":{\"connectorIds\":[],\"side\":\"TOP\"},\"type\":\"ConnectorPlacement.EquallySpacedRectSide\",\"uuid\":\"06046061-3240-493e-a0a3-282c9541adae\"}]},\"type\":\"ConnectorPlacement.EquallySpacedConnector\",\"uuid\":\"b0591291-fd4b-4355-beaa-e569a19c4b12\"}],\"packageUris\":[\"http://schema.mathworks.com/mf0/Connector/R2020b\"],\"version\":\"1.0\"}"
  MixtureVolume : Gain  Gain=Volume
  String Constant : StringConstant  String="\"upwards\""
  Subsystem : Subsystem  ReferencedSubsystem=kCalculation
      settings: PortSchema="{\"entries\":[{\"content\":{\"sides\":[{\"content\":{\"connectorIds\":[\"In2\",\"In3\",\"In4\",\"In5\",\"In6\",\"In7\",\"In1\"]},\"type\":\"ConnectorPlacement.EquallySpacedRectSide\",\"uuid\":\"002a6616-4b3b-4d3e-9efd-a784f6bbe134\"},{\"content\":{\"connectorIds\":[\"Out1\",\"Out2\"],\"side\":\"RIGHT\"},\"type\":\"ConnectorPlacement.EquallySpacedRectSide\",\"uuid\":\"da6acc14-6515-461b-8149-f4cbf493a4dd\"},{\"content\":{\"connectorIds\":[],\"side\":\"TOP\"},\"type\":\"ConnectorPlacement.EquallySpacedRectSide\",\"uuid\":\"939e49a4-f3cd-4ed3-a7a5-6bbefe0ae08a\"},{\"content\":{\"connectorIds\":[\"In8\"],\"side\":\"BOTTOM\"},\"type\":\"ConnectorPlacement.EquallySpacedRectSide\",\"uuid\":\"3faad216-807b-414f-aa2c-73b0ff13b323\"}]},\"type\":\"ConnectorPlacement.EquallySpacedConnector\",\"uuid\":\"8f0c794e-eb76-47c6-abaf-8e07cad1f307\"}],\"packageUris\":[\"http://schema.mathworks.com/mf0/Connector/R2020b\"],\"version\":\"1.0\"}"
  Subsystem1 : Subsystem  ReferencedSubsystem=GasToAlpha
  Transfer Term : MATLAB Function  TreatAsAtomicUnit=on
  Ref : PMIOPort  Side=Left
  TranfserRate : Outport
  wires:
  Transfer Term/1(volRate) -> MixtureVolume/1
  MixtureVolume/1 -> TranfserRate/1
  VolumeRate/1 -> Constitutive/3(VolumeRate)
  GasRef/1 -> Subsystem1/1
  Subsystem1/1 -> Constitutive/1(alpha), Transfer Term/3(alpha)
  Constitutive/1(ul) -> Transfer Term/4(ul)
  Constitutive/2(ug) -> Transfer Term/5(ug)
  Constant/1 -> Subsystem/7, Constitutive/4(Diam)
  GxSalt/1 -> Transfer Term/1(GxS)
  GxGas/1 -> Transfer Term/2(GxG)
  Subsystem/1 -> Transfer Term/7(dsm)
  Subsystem/2 -> Transfer Term/8(k)
  PLoss/1 -> Constitutive/2(PLoss)
  Constitutive/4(Re) -> Subsystem/2
  Constitutive/3(K) -> Transfer Term/6(K)
  Constitutive/5(Sc) -> Subsystem/3
  Constitutive/6(Diff) -> Subsystem/4
  Constitutive/7(alphaC) -> Subsystem/5
  Constitutive/8(dsm) -> Subsystem/6
  Constitutive/9(f_m) -> Subsystem/1
  String Constant/1 -> Subsystem/8
  connections:
  Constitutive/LConn1 -- Ref/RConn1

== system MSDRPrimaryLoop/Reactor/CoreTH&Inerti/UpperPlenum/XenonCalc/Salt ==
  XeLIn : Inport  PortDimensions=1
  IodineSNumberDensity : Inport  Port=2  PortDimensions=1
  T_f_ave : Inport  Port=3
  GasRef : Inport  Port=4  PortDimensions=1
  VolumeRate : Inport  Port=5
  Interphase : Inport  Port=6
  Add : Sum  Inputs=+++--  InputSameDT=on
  Add1 : Sum
  Decay : Gain  Gain=xeDecayConstant
  Gain1 : Gain  Gain=0.5/Area
  InPipeGeneration : Subsystem
      settings: PortSchema="{\"entries\":[{\"content\":{\"sides\":[{\"content\":{\"connectorIds\":[\"In1\"]},\"type\":\"ConnectorPlacement.EquallySpacedRectSide\",\"uuid\":\"cf58f9e2-4051-4ec0-bfd5-a375f3464f67\"},{\"content\":{\"connectorIds\":[\"Out1\"],\"side\":\"RIGHT\"},\"type\":\"ConnectorPlacement.EquallySpacedRectSide\",\"uuid\":\"cf475b22-0422-4ebc-b148-ab559744c6ba\"},{\"content\":{\"connectorIds\":[],\"side\":\"TOP\"},\"type\":\"ConnectorPlacement.EquallySpacedRectSide\",\"uuid\":\"15cc78ce-ee79-4f49-b098-b77c0b2a8ba1\"},{\"content\":{\"connectorIds\":[\"In2\"],\"side\":\"BOTTOM\"},\"type\":\"ConnectorPlacement.EquallySpacedRectSide\",\"uuid\":\"64f5be1f-19d6-4b5f-ac24-c41659a6a539\"}]},\"type\":\"ConnectorPlacement.EquallySpacedConnector\",\"uuid\":\"1fb1607a-ceed-4d70-a511-7b706be0d7ea\"}],\"packageUris\":[\"http://schema.mathworks.com/mf0/Connector/R2020b\"],\"version\":\"1.0\"}"
  LiquidFlowRate : Product
  LiquidVolume : Product  Inputs=*/
  MixtureVolume : Gain  Gain=1/Volume
  PhaseMass : Integrator  LimitOutput=on  LowerSaturationLimit=0
  Subsystem1 : Subsystem
  XeLOut : Outport  PortDimensions=1
  GxSalt : Outport  Port=2
  wires:
  LiquidFlowRate/1 -> Add/5, XeLOut/1, Add1/2
  IodineSNumberDensity/1 -> InPipeGeneration/1(IodineSNumberDensity)
  LiquidVolume/1 -> LiquidFlowRate/2
  Add/1 -> PhaseMass/1
  MixtureVolume/1 -> LiquidVolume/1
  VolumeRate/1 -> LiquidFlowRate/1
  T_f_ave/1 -> InPipeGeneration/2(T_f_ave)
  PhaseMass/1 -> Decay/1, MixtureVolume/1
  GasRef/1 -> Subsystem1/1(Gas)
  Subsystem1/1(1-alpha) -> LiquidVolume/2
  InPipeGeneration/1("XenonGenerationRate, [kg/s]") -> Add/2
  XeLIn/1 -> Add1/1, Add/1
  Add1/1 -> Gain1/1
  Gain1/1 -> GxSalt/1
  Interphase/1 -> Add/3
  Decay/1 -> Add/4

== system MSDRPrimaryLoop/Reactor/Reactivity&PKE/Reactivity&PKE/Xe and Sm/Samarium ==
  NeutronFraction : Inport
  BurnUp : Product
  InCoreFraction : Gain  Gain=V_reactor_fuel/(V_reactor_fuel + V_primary_fuel)
  IncoreCrossSection : Gain  Gain=sigma_sm149
  Nd149/Pm149Yield : Constant  Value=Nd149Yield
  NominalFissionRate : Constant  Value=NominalFissionRate
  NominalFlux : Constant  Value=NominalFlux
  PmAtoms : Integrator  InitialCondition=NominalFissionRate*Nd149Yield/PmDecayConstant
  PmDecay : Gain  Gain=PmDecayConstant
  "PmGeneration, [1/s]" : Product
  Product : Product
  Product1 : Product
  SMAtoms1 : Integrator  InitialCondition=NominalFissionRate*Nd149Yield/(NominalFlux*sigma_sm149)*(V_reactor_fuel + V_primary_fuel)/V_reactor_fuel
  Sum : Sum  Inputs=|+-
  Sum1 : Sum  Inputs=+-
  "SmInCore, [cm2]" : Outport
  wires:
  NeutronFraction/1 -> Product/1, Product1/1
  NominalFissionRate/1 -> Product/2
  Product/1 -> "PmGeneration, [1/s]"/1
  Nd149/Pm149Yield/1 -> "PmGeneration, [1/s]"/2
  "PmGeneration, [1/s]"/1 -> Sum/1
  Sum/1 -> PmAtoms/1
  PmAtoms/1 -> PmDecay/1
  PmDecay/1 -> Sum1/1, Sum/2
  Sum1/1 -> SMAtoms1/1
  NominalFlux/1 -> Product1/2
  Product1/1 -> BurnUp/1
  InCoreFraction/1 -> IncoreCrossSection/1
  SMAtoms1/1 -> InCoreFraction/1
  IncoreCrossSection/1 -> "SmInCore, [cm2]"/1, BurnUp/2
  BurnUp/1 -> Sum1/2

== system MSDRPrimaryLoop/Chemical Processing/Bubble Generator/XenonCalc/InterphaseTranfser/Constitutive/Subsystem ==
  note: Specific for Bubble Generator
  note: Include the form loss to averaged frictional factor as a rough estimate.
  PLoss : Inport
  Dh : Inport  Port=2
  ul : Inport  Port=3
  Constant2 : Constant  Value=Dsm
  Divide : Product  Inputs=**//
  Gain : Gain  Gain=2/Length
  Math Function : Math  Operator=square  SaturateOnIntegerOverflow=on
  PS-Simulink Converter : nesl_utility/PS-Simulink Converter  PhysicalDomain=network_engine_domain  SubClassName=ps_output  LeftPortType=input  RightPortType=output  PseudoPeriodic=off  Frequencies=[]  Unit=inherit  AffineConversion=off
      settings: SourceProductBaseCode=PW,SS
  Simscape Component : SimscapeComponentBlock  SourceFile=TL_FullSensor  ComponentPath=TL_FullSensor  ComponentVariants="[\"TL_FullSensor\"]"  ComponentVariantNames="[\"TL_FullSensor\"]"  ClassName=TL_FullSensor  SchemaVersion=1
      settings: CopyFcn=simscape.engine.sli.internal.componentblockcallback(gcbh,'COPY')  PreCopyFcn=simscape.engine.sli.internal.componentblockcallback(gcbh,'PRECOPY')  PreDeleteFcn=simscape.engine.sli.internal.componentblockcallback(gcbh,'PREDELETE')  InternalSimscapePortConfiguration="{\"Bottom\":[],\"Left\":[{\"id\":\"A\",\"label\":\"A\",\"type\":\"foundation.thermal_liquid.thermal_liquid\"}],\"Right\":[{\"id\":\"U\",\"label\":\"u\",\"type\":\"output\"},{\"id\":\"RHO\",\"label\":\"rho\",\"type\":\"output\"},{\"id\":\"CP\",\"label\":\"cp\",\"type\":\"output\"},{\"id\":\"NU\",\"label\":\"nu\",\"type\":\"output\"}],\"Top\":[]}"
      mask Type: Thermodynamic Properties Sensor (TL)
      mask Display: color('red');plot([0 1 1 0 0],[0 0 1 1 0]);plot([0.7,1],[1,0.7]);plot(-2,-1.75);plot(3, 1);disp('\n.ssc\nUnresolved')
  Ref : PMIOPort  Side=Right
  f_Combined : Outport
  dsm : Outport  Port=2
  wires:
  Dh/1 -> Divide/2
  Divide/1 -> f_Combined/1
  Math Function/1 -> Divide/3
  Constant2/1 -> dsm/1
  ul/1 -> Math Function/1
  PS-Simulink Converter/1 -> Divide/4
  Gain/1 -> Divide/1
  PLoss/1 -> Gain/1
  connections:
  Simscape Component/LConn1 -- Ref/RConn1
  Simscape Component/RConn2 -- PS-Simulink Converter/LConn1

== system MSDRPrimaryLoop/Chemical Processing/ElevationPipe/XenonCalc/InterphaseTranfser1/Constitutive/Subsystem ==
  note: Calculation of Dsm in the pipeLine is a complicated problem. In a long pipeline, it is expected that coalescence will happen. A small bubble diameter is not physically possible to be maintained over a signicant length and void fraction.
      |
      | For sake of the analysis, the constant value is used. However, it now should only be thought as an averaged value between dcr and din.
      | Extreme small imput of bubble diameter is to be avoided.
      |
      | This is at least a 1D transport equation problem that I'm not willing to take at this moment.
  note: Include the form loss to averaged frictional factor as a rough estimate.
  PLoss : Inport
  Dh : Inport  Port=2
  ul : Inport  Port=3
  Constant2 : Constant  Value=generatorDsm
  Divide : Product  Inputs=**//
  Gain : Gain  Gain=2/Length
  Math Function : Math  Operator=square  SaturateOnIntegerOverflow=on
  PS-Simulink Converter : nesl_utility/PS-Simulink Converter  PhysicalDomain=network_engine_domain  SubClassName=ps_output  LeftPortType=input  RightPortType=output  PseudoPeriodic=off  Frequencies=[]  Unit=inherit  AffineConversion=off
      settings: SourceProductBaseCode=PW,SS
  Simscape Component : SimscapeComponentBlock  SourceFile=TL_FullSensor  ComponentPath=TL_FullSensor  ComponentVariants="[\"TL_FullSensor\"]"  ComponentVariantNames="[\"TL_FullSensor\"]"  ClassName=TL_FullSensor  SchemaVersion=1
      settings: CopyFcn=simscape.engine.sli.internal.componentblockcallback(gcbh,'COPY')  PreCopyFcn=simscape.engine.sli.internal.componentblockcallback(gcbh,'PRECOPY')  PreDeleteFcn=simscape.engine.sli.internal.componentblockcallback(gcbh,'PREDELETE')  InternalSimscapePortConfiguration="{\"Bottom\":[],\"Left\":[{\"id\":\"A\",\"label\":\"A\",\"type\":\"foundation.thermal_liquid.thermal_liquid\"}],\"Right\":[{\"id\":\"U\",\"label\":\"u\",\"type\":\"output\"},{\"id\":\"RHO\",\"label\":\"rho\",\"type\":\"output\"},{\"id\":\"CP\",\"label\":\"cp\",\"type\":\"output\"},{\"id\":\"NU\",\"label\":\"nu\",\"type\":\"output\"}],\"Top\":[]}"
      mask Type: Thermodynamic Properties Sensor (TL)
  Ref : PMIOPort  Side=Right
  f_Combined : Outport
  dsm : Outport  Port=2
  wires:
  Dh/1 -> Divide/2
  Divide/1 -> f_Combined/1
  Math Function/1 -> Divide/3
  Constant2/1 -> dsm/1
  ul/1 -> Math Function/1
  PS-Simulink Converter/1 -> Divide/4
  Gain/1 -> Divide/1
  PLoss/1 -> Gain/1
  connections:
  Simscape Component/LConn1 -- Ref/RConn1
  Simscape Component/RConn2 -- PS-Simulink Converter/LConn1

== system MSDRPrimaryLoop/Chemical Processing/PipeLine/XenonCalc/InterphaseTranfser/Constitutive/Subsystem ==
  note: Calculation of Dsm in the pipeLine is a complicated problem. In a long pipeline, it is expected that coalescence will happen. A small bubble diameter is not physically possible to be maintained over a signicant length and void fraction.
      |
      | For sake of the analysis, the constant value is used. However, it now should only be thought as an averaged value between dcr and din.
      | Extreme small imput of bubble diameter is to be avoided.
      |
      | This is at least a 1D transport equation problem that I'm not willing to take at this moment.
      | I could put in the same equation I used to blend the dsm in core. But I'm not really proud of that one.
      |
      | A problem requires a bit more discussion with Prof. Brooks.
  note: Include the form loss to averaged frictional factor as a rough estimate.
  PLoss : Inport
  Dh : Inport  Port=2
  ul : Inport  Port=3
  Constant2 : Constant  Value=Dsm
  Divide : Product  Inputs=**//
  Gain : Gain  Gain=2/Length
  Math Function : Math  Operator=square  SaturateOnIntegerOverflow=on
  PS-Simulink Converter : nesl_utility/PS-Simulink Converter  PhysicalDomain=network_engine_domain  SubClassName=ps_output  LeftPortType=input  RightPortType=output  PseudoPeriodic=off  Frequencies=[]  Unit=inherit  AffineConversion=off
      settings: SourceProductBaseCode=PW,SS
  Simscape Component : SimscapeComponentBlock  SourceFile=TL_FullSensor  ComponentPath=TL_FullSensor  ComponentVariants="[\"TL_FullSensor\"]"  ComponentVariantNames="[\"TL_FullSensor\"]"  ClassName=TL_FullSensor  SchemaVersion=1
      settings: CopyFcn=simscape.engine.sli.internal.componentblockcallback(gcbh,'COPY')  PreCopyFcn=simscape.engine.sli.internal.componentblockcallback(gcbh,'PRECOPY')  PreDeleteFcn=simscape.engine.sli.internal.componentblockcallback(gcbh,'PREDELETE')  InternalSimscapePortConfiguration="{\"Bottom\":[],\"Left\":[{\"id\":\"A\",\"label\":\"A\",\"type\":\"foundation.thermal_liquid.thermal_liquid\"}],\"Right\":[{\"id\":\"U\",\"label\":\"u\",\"type\":\"output\"},{\"id\":\"RHO\",\"label\":\"rho\",\"type\":\"output\"},{\"id\":\"CP\",\"label\":\"cp\",\"type\":\"output\"},{\"id\":\"NU\",\"label\":\"nu\",\"type\":\"output\"}],\"Top\":[]}"
      mask Type: Thermodynamic Properties Sensor (TL)
      mask Display: color('red');plot([0 1 1 0 0],[0 0 1 1 0]);plot([0.7,1],[1,0.7]);plot(-2,-1.75);plot(3, 1);disp('\n.ssc\nUnresolved')
  Ref : PMIOPort  Side=Right
  f_Combined : Outport
  dsm : Outport  Port=2
  wires:
  Dh/1 -> Divide/2
  Divide/1 -> f_Combined/1
  Math Function/1 -> Divide/3
  Constant2/1 -> dsm/1
  ul/1 -> Math Function/1
  PS-Simulink Converter/1 -> Divide/4
  Gain/1 -> Divide/1
  PLoss/1 -> Gain/1
  connections:
  Simscape Component/LConn1 -- Ref/RConn1
  Simscape Component/RConn2 -- PS-Simulink Converter/LConn1
